simulink model "slide_6_model"  (R2026a)
settings: Solver=VariableStepAuto
values from neighbouring files (symbols this model uses):
  b = 0.2    [ode45.mat]
  k = 1    [ode45.mat]
  m = 1    [ode45.mat]
undefined symbols (not defined in the file or in its folder): Ft
settings Model: Creator=tdxt  LastModifiedBy=tdxt

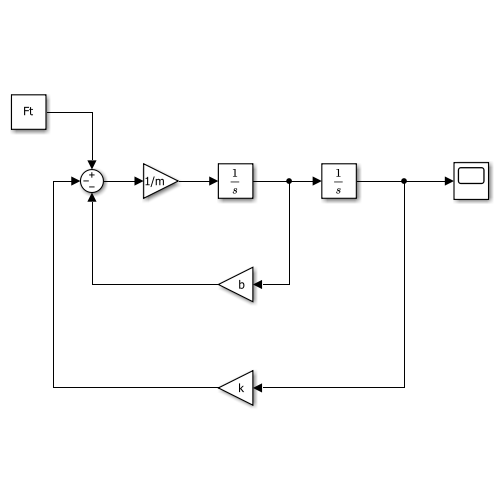
[thumbnail: Simulink's stored preview of the top-level diagram]
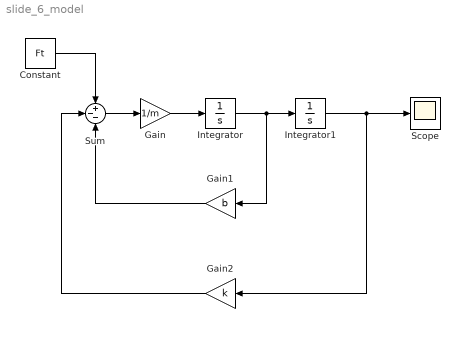
== system slide_6_model ==
  Constant : Constant  Value=Ft
  Gain : Gain  Gain=1/m
  Gain1 : Gain  Gain=b
  Gain2 : Gain  Gain=k
  Integrator : Integrator
  Integrator1 : Integrator  InitialCondition=1
  Scope : Scope
  Sum : Sum  Inputs=+--
  wires:
  Sum/1 -> Gain/1
  Gain/1 -> Integrator/1
  Integrator/1 -> Gain1/1, Integrator1/1
  Integrator1/1 -> Gain2/1, Scope/1
  Gain2/1 -> Sum/2
  Gain1/1 -> Sum/3
  Constant/1 -> Sum/1
